simulink model "simple_router"  (R2015a)
settings: Solver=ode45  StartTime=0.0  StopTime=3000  FixedStep=1  RelTol=1e-3
undefined symbols (not defined in the file or in its folder): des, SELECT, T
libraries: simulink x16
(part 3 of 6)

== system simple_router/Router01 ==
  Attribute Function : Subsystem  LoadFcn=des.afb.attributefunction_support(gcb,'LoadFcn');  StartFcn=des.afb.attributefunction_support(gcb,'StartFcn');  mask(Attribute Function){OutputNamePrefix=out_}
      mask prompts: OutputNamePrefix "Prefix name"
      settings: CopyFcn=des.afb.attributefunction_support(gcb,'CopyFcn');  OpenFcn=des.afb.attributefunction_support(gcb,'OpenFcn');  ErrorFcn=des.afb.error_redirect
      mask Help: slhelp(gcbh)
      mask Display: image(des_iconLoad('attribFunction.jpg'),'center');
  Clocked FIFO1 : Subsystem  mask{E=1/F, S=S, F=C}
      mask prompts: E "Clock Period (s)"; S "Standard Deviation"; F "FIFO capacity"
  Clocked FIFO2 : Subsystem  mask{E=1, S=.1, F=8}
      mask prompts: E "Clock Period (s)"; S "Standard Deviation"; F "FIFO capacity"
  Clocked FIFO3 : Subsystem  mask{E=1, S=.1, F=8}
      mask prompts: E "Clock Period (s)"; S "Standard Deviation"; F "FIFO capacity"
  Clocked FIFO4 : Subsystem  mask{E=1, S=.1, F=8}
      mask prompts: E "Clock Period (s)"; S "Standard Deviation"; F "FIFO capacity"
  Clocked FIFO5 : Subsystem  mask{E=1, S=.1, F=8}
      mask prompts: E "Clock Period (s)"; S "Standard Deviation"; F "FIFO capacity"
  Constant : Constant  Value=ME
  Output Switch1 : OutputSwitch  NumberOutputPorts=5  SwitchingCriterion=From attribute  AttributeName=RT  InitialConditionsOpt=on  InitialConditions=5
  Path Combiner : PathCombiner  NumberInputPorts=5  InputPortPrecedence=Equiprobable  InitialSeed=2
  Set Attribute : SetAttribute  AttributeName=ME  AttributeFrom=Signal port  EvaluatedAttributeValue={ []}
  Single Server1 : SingleServer  ServiceTime=D
  DataOut_N : PMIOPort  Port=1  Side=Left
  DataIn_N : PMIOPort  Port=2  Side=Right
  DataIn_W : PMIOPort  Port=3  Side=Left
  DataOut_W : PMIOPort  Port=4  Side=Right
  DataIn_E : PMIOPort  Port=5  Side=Left
  DataOut_E : PMIOPort  Port=6  Side=Right
  DataIn_S : PMIOPort  Port=7  Side=Left
  DataOut_S : PMIOPort  Port=8  Side=Right
  DataIn_NI : PMIOPort  Port=9  Side=Left
  DataOut_NI : PMIOPort  Port=10  Side=Right
  wires:
  Constant/1 -> Set Attribute/1
  connections:
  DataIn_W/RConn1 -- Clocked FIFO2/LConn1
  Clocked FIFO4/LConn1 -- DataIn_E/RConn1
  Clocked FIFO3/LConn1 -- DataIn_S/RConn1
  DataIn_N/RConn1 -- Clocked FIFO1/LConn1
  Clocked FIFO5/LConn1 -- DataIn_NI/RConn1
  Set Attribute/RConn1 -- Attribute Function/LConn1
  Output Switch1/LConn1 -- Single Server1/RConn1
  Single Server1/LConn1 -- Attribute Function/RConn1
  Path Combiner/RConn1 -- Set Attribute/LConn1
  Clocked FIFO1/RConn1 -- Path Combiner/LConn1
  Clocked FIFO2/RConn1 -- Path Combiner/LConn2
  Clocked FIFO4/RConn1 -- Path Combiner/LConn3
  Clocked FIFO3/RConn1 -- Path Combiner/LConn4
  Clocked FIFO5/RConn1 -- Path Combiner/LConn5
  DataOut_N/RConn1 -- Output Switch1/RConn1
  DataOut_W/RConn1 -- Output Switch1/RConn2
  DataOut_E/RConn1 -- Output Switch1/RConn3
  DataOut_S/RConn1 -- Output Switch1/RConn4
  DataOut_NI/RConn1 -- Output Switch1/RConn5

== system simple_router/Router02 ==
  Attribute Function : Subsystem  LoadFcn=des.afb.attributefunction_support(gcb,'LoadFcn');  StartFcn=des.afb.attributefunction_support(gcb,'StartFcn');  mask(Attribute Function){OutputNamePrefix=out_}
      mask prompts: OutputNamePrefix "Prefix name"
      settings: CopyFcn=des.afb.attributefunction_support(gcb,'CopyFcn');  OpenFcn=des.afb.attributefunction_support(gcb,'OpenFcn');  ErrorFcn=des.afb.error_redirect
      mask Help: slhelp(gcbh)
      mask Display: image(des_iconLoad('attribFunction.jpg'),'center');
  Clocked FIFO1 : Subsystem  mask{E=1/F, S=S, F=C}
      mask prompts: E "Clock Period (s)"; S "Standard Deviation"; F "FIFO capacity"
  Clocked FIFO2 : Subsystem  mask{E=1, S=.1, F=8}
      mask prompts: E "Clock Period (s)"; S "Standard Deviation"; F "FIFO capacity"
  Clocked FIFO3 : Subsystem  mask{E=1, S=.1, F=8}
      mask prompts: E "Clock Period (s)"; S "Standard Deviation"; F "FIFO capacity"
  Clocked FIFO4 : Subsystem  mask{E=1, S=.1, F=8}
      mask prompts: E "Clock Period (s)"; S "Standard Deviation"; F "FIFO capacity"
  Clocked FIFO5 : Subsystem  mask{E=1, S=.1, F=8}
      mask prompts: E "Clock Period (s)"; S "Standard Deviation"; F "FIFO capacity"
  Constant : Constant  Value=ME
  Output Switch1 : OutputSwitch  NumberOutputPorts=5  SwitchingCriterion=From attribute  AttributeName=RT  InitialConditionsOpt=on  InitialConditions=5
  Path Combiner : PathCombiner  NumberInputPorts=5  InputPortPrecedence=Equiprobable  InitialSeed=2
  Set Attribute : SetAttribute  AttributeName=ME  AttributeFrom=Signal port  EvaluatedAttributeValue={ []}
  Single Server1 : SingleServer  ServiceTime=D
  DataOut_N : PMIOPort  Port=1  Side=Left
  DataIn_N : PMIOPort  Port=2  Side=Right
  DataIn_W : PMIOPort  Port=3  Side=Left
  DataOut_W : PMIOPort  Port=4  Side=Right
  DataIn_E : PMIOPort  Port=5  Side=Left
  DataOut_E : PMIOPort  Port=6  Side=Right
  DataIn_S : PMIOPort  Port=7  Side=Left
  DataOut_S : PMIOPort  Port=8  Side=Right
  DataIn_NI : PMIOPort  Port=9  Side=Left
  DataOut_NI : PMIOPort  Port=10  Side=Right
  wires:
  Constant/1 -> Set Attribute/1
  connections:
  DataIn_W/RConn1 -- Clocked FIFO2/LConn1
  Clocked FIFO4/LConn1 -- DataIn_E/RConn1
  Clocked FIFO3/LConn1 -- DataIn_S/RConn1
  DataIn_N/RConn1 -- Clocked FIFO1/LConn1
  Clocked FIFO5/LConn1 -- DataIn_NI/RConn1
  Set Attribute/RConn1 -- Attribute Function/LConn1
  Output Switch1/LConn1 -- Single Server1/RConn1
  Single Server1/LConn1 -- Attribute Function/RConn1
  Path Combiner/RConn1 -- Set Attribute/LConn1
  Clocked FIFO1/RConn1 -- Path Combiner/LConn1
  Clocked FIFO2/RConn1 -- Path Combiner/LConn2
  Clocked FIFO4/RConn1 -- Path Combiner/LConn3
  Clocked FIFO3/RConn1 -- Path Combiner/LConn4
  Clocked FIFO5/RConn1 -- Path Combiner/LConn5
  DataOut_N/RConn1 -- Output Switch1/RConn1
  DataOut_W/RConn1 -- Output Switch1/RConn2
  DataOut_E/RConn1 -- Output Switch1/RConn3
  DataOut_S/RConn1 -- Output Switch1/RConn4
  DataOut_NI/RConn1 -- Output Switch1/RConn5

== system simple_router/Router03 ==
  Attribute Function : Subsystem  LoadFcn=des.afb.attributefunction_support(gcb,'LoadFcn');  StartFcn=des.afb.attributefunction_support(gcb,'StartFcn');  mask(Attribute Function){OutputNamePrefix=out_}
      mask prompts: OutputNamePrefix "Prefix name"
      settings: CopyFcn=des.afb.attributefunction_support(gcb,'CopyFcn');  OpenFcn=des.afb.attributefunction_support(gcb,'OpenFcn');  ErrorFcn=des.afb.error_redirect
      mask Help: slhelp(gcbh)
      mask Display: image(des_iconLoad('attribFunction.jpg'),'center');
  Clocked FIFO1 : Subsystem  mask{E=1/F, S=S, F=C}
      mask prompts: E "Clock Period (s)"; S "Standard Deviation"; F "FIFO capacity"
  Clocked FIFO2 : Subsystem  mask{E=1, S=.1, F=8}
      mask prompts: E "Clock Period (s)"; S "Standard Deviation"; F "FIFO capacity"
  Clocked FIFO3 : Subsystem  mask{E=1, S=.1, F=8}
      mask prompts: E "Clock Period (s)"; S "Standard Deviation"; F "FIFO capacity"
  Clocked FIFO4 : Subsystem  mask{E=1, S=.1, F=8}
      mask prompts: E "Clock Period (s)"; S "Standard Deviation"; F "FIFO capacity"
  Clocked FIFO5 : Subsystem  mask{E=1, S=.1, F=8}
      mask prompts: E "Clock Period (s)"; S "Standard Deviation"; F "FIFO capacity"
  Constant : Constant  Value=ME
  Output Switch1 : OutputSwitch  NumberOutputPorts=5  SwitchingCriterion=From attribute  AttributeName=RT  InitialConditionsOpt=on  InitialConditions=5
  Path Combiner : PathCombiner  NumberInputPorts=5  InputPortPrecedence=Equiprobable  InitialSeed=2
  Set Attribute : SetAttribute  AttributeName=ME  AttributeFrom=Signal port  EvaluatedAttributeValue={ []}
  Single Server1 : SingleServer  ServiceTime=D
  DataOut_N : PMIOPort  Port=1  Side=Left
  DataIn_N : PMIOPort  Port=2  Side=Right
  DataIn_W : PMIOPort  Port=3  Side=Left
  DataOut_W : PMIOPort  Port=4  Side=Right
  DataIn_E : PMIOPort  Port=5  Side=Left
  DataOut_E : PMIOPort  Port=6  Side=Right
  DataIn_S : PMIOPort  Port=7  Side=Left
  DataOut_S : PMIOPort  Port=8  Side=Right
  DataIn_NI : PMIOPort  Port=9  Side=Left
  DataOut_NI : PMIOPort  Port=10  Side=Right
  wires:
  Constant/1 -> Set Attribute/1
  connections:
  DataIn_W/RConn1 -- Clocked FIFO2/LConn1
  Clocked FIFO4/LConn1 -- DataIn_E/RConn1
  Clocked FIFO3/LConn1 -- DataIn_S/RConn1
  DataIn_N/RConn1 -- Clocked FIFO1/LConn1
  Clocked FIFO5/LConn1 -- DataIn_NI/RConn1
  Set Attribute/RConn1 -- Attribute Function/LConn1
  Output Switch1/LConn1 -- Single Server1/RConn1
  Single Server1/LConn1 -- Attribute Function/RConn1
  Path Combiner/RConn1 -- Set Attribute/LConn1
  Clocked FIFO1/RConn1 -- Path Combiner/LConn1
  Clocked FIFO2/RConn1 -- Path Combiner/LConn2
  Clocked FIFO4/RConn1 -- Path Combiner/LConn3
  Clocked FIFO3/RConn1 -- Path Combiner/LConn4
  Clocked FIFO5/RConn1 -- Path Combiner/LConn5
  DataOut_N/RConn1 -- Output Switch1/RConn1
  DataOut_W/RConn1 -- Output Switch1/RConn2
  DataOut_E/RConn1 -- Output Switch1/RConn3
  DataOut_S/RConn1 -- Output Switch1/RConn4
  DataOut_NI/RConn1 -- Output Switch1/RConn5

== system simple_router/Router09 ==
  Attribute Function : Subsystem  LoadFcn=des.afb.attributefunction_support(gcb,'LoadFcn');  StartFcn=des.afb.attributefunction_support(gcb,'StartFcn');  mask(Attribute Function){OutputNamePrefix=out_}
      mask prompts: OutputNamePrefix "Prefix name"
      settings: CopyFcn=des.afb.attributefunction_support(gcb,'CopyFcn');  OpenFcn=des.afb.attributefunction_support(gcb,'OpenFcn');  ErrorFcn=des.afb.error_redirect
      mask Help: slhelp(gcbh)
      mask Display: image(des_iconLoad('attribFunction.jpg'),'center');
  Clocked FIFO1 : Subsystem  mask{E=1/F, S=S, F=C}
      mask prompts: E "Clock Period (s)"; S "Standard Deviation"; F "FIFO capacity"
  Clocked FIFO2 : Subsystem  mask{E=1, S=.1, F=8}
      mask prompts: E "Clock Period (s)"; S "Standard Deviation"; F "FIFO capacity"
  Clocked FIFO3 : Subsystem  mask{E=1, S=.1, F=8}
      mask prompts: E "Clock Period (s)"; S "Standard Deviation"; F "FIFO capacity"
  Clocked FIFO4 : Subsystem  mask{E=1, S=.1, F=8}
      mask prompts: E "Clock Period (s)"; S "Standard Deviation"; F "FIFO capacity"
  Clocked FIFO5 : Subsystem  mask{E=1, S=.1, F=8}
      mask prompts: E "Clock Period (s)"; S "Standard Deviation"; F "FIFO capacity"
  Constant : Constant  Value=ME
  Output Switch1 : OutputSwitch  NumberOutputPorts=5  SwitchingCriterion=From attribute  AttributeName=RT  InitialConditionsOpt=on  InitialConditions=5
  Path Combiner : PathCombiner  NumberInputPorts=5  InputPortPrecedence=Equiprobable  InitialSeed=2
  Set Attribute : SetAttribute  AttributeName=ME  AttributeFrom=Signal port  EvaluatedAttributeValue={ []}
  Single Server1 : SingleServer  ServiceTime=D
  DataOut_N : PMIOPort  Port=1  Side=Left
  DataIn_N : PMIOPort  Port=2  Side=Right
  DataIn_W : PMIOPort  Port=3  Side=Left
  DataOut_W : PMIOPort  Port=4  Side=Right
  DataIn_E : PMIOPort  Port=5  Side=Left
  DataOut_E : PMIOPort  Port=6  Side=Right
  DataIn_S : PMIOPort  Port=7  Side=Left
  DataOut_S : PMIOPort  Port=8  Side=Right
  DataIn_NI : PMIOPort  Port=9  Side=Left
  DataOut_NI : PMIOPort  Port=10  Side=Right
  wires:
  Constant/1 -> Set Attribute/1
  connections:
  DataIn_W/RConn1 -- Clocked FIFO2/LConn1
  Clocked FIFO4/LConn1 -- DataIn_E/RConn1
  Clocked FIFO3/LConn1 -- DataIn_S/RConn1
  DataIn_N/RConn1 -- Clocked FIFO1/LConn1
  Clocked FIFO5/LConn1 -- DataIn_NI/RConn1
  Set Attribute/RConn1 -- Attribute Function/LConn1
  Output Switch1/LConn1 -- Single Server1/RConn1
  Single Server1/LConn1 -- Attribute Function/RConn1
  Path Combiner/RConn1 -- Set Attribute/LConn1
  Clocked FIFO1/RConn1 -- Path Combiner/LConn1
  Clocked FIFO2/RConn1 -- Path Combiner/LConn2
  Clocked FIFO4/RConn1 -- Path Combiner/LConn3
  Clocked FIFO3/RConn1 -- Path Combiner/LConn4
  Clocked FIFO5/RConn1 -- Path Combiner/LConn5
  DataOut_N/RConn1 -- Output Switch1/RConn1
  DataOut_W/RConn1 -- Output Switch1/RConn2
  DataOut_E/RConn1 -- Output Switch1/RConn3
  DataOut_S/RConn1 -- Output Switch1/RConn4
  DataOut_NI/RConn1 -- Output Switch1/RConn5

== system simple_router/Router10 ==
  Attribute Function : Subsystem  LoadFcn=des.afb.attributefunction_support(gcb,'LoadFcn');  StartFcn=des.afb.attributefunction_support(gcb,'StartFcn');  mask(Attribute Function){OutputNamePrefix=out_}
      mask prompts: OutputNamePrefix "Prefix name"
      settings: CopyFcn=des.afb.attributefunction_support(gcb,'CopyFcn');  OpenFcn=des.afb.attributefunction_support(gcb,'OpenFcn');  ErrorFcn=des.afb.error_redirect
      mask Help: slhelp(gcbh)
      mask Display: image(des_iconLoad('attribFunction.jpg'),'center');
  Clocked FIFO1 : Subsystem  mask{E=1/F, S=S, F=C}
      mask prompts: E "Clock Period (s)"; S "Standard Deviation"; F "FIFO capacity"
  Clocked FIFO2 : Subsystem  mask{E=1, S=.1, F=8}
      mask prompts: E "Clock Period (s)"; S "Standard Deviation"; F "FIFO capacity"
  Clocked FIFO3 : Subsystem  mask{E=1, S=.1, F=8}
      mask prompts: E "Clock Period (s)"; S "Standard Deviation"; F "FIFO capacity"
  Clocked FIFO4 : Subsystem  mask{E=1, S=.1, F=8}
      mask prompts: E "Clock Period (s)"; S "Standard Deviation"; F "FIFO capacity"
  Clocked FIFO5 : Subsystem  mask{E=1, S=.1, F=8}
      mask prompts: E "Clock Period (s)"; S "Standard Deviation"; F "FIFO capacity"
  Constant : Constant  Value=ME
  Output Switch1 : OutputSwitch  NumberOutputPorts=5  SwitchingCriterion=From attribute  AttributeName=RT  InitialConditionsOpt=on  InitialConditions=5
  Path Combiner : PathCombiner  NumberInputPorts=5  InputPortPrecedence=Equiprobable  InitialSeed=2
  Set Attribute : SetAttribute  AttributeName=ME  AttributeFrom=Signal port  EvaluatedAttributeValue={ []}
  Single Server1 : SingleServer  ServiceTime=D
  DataOut_N : PMIOPort  Port=1  Side=Left
  DataIn_N : PMIOPort  Port=2  Side=Right
  DataIn_W : PMIOPort  Port=3  Side=Left
  DataOut_W : PMIOPort  Port=4  Side=Right
  DataIn_E : PMIOPort  Port=5  Side=Left
  DataOut_E : PMIOPort  Port=6  Side=Right
  DataIn_S : PMIOPort  Port=7  Side=Left
  DataOut_S : PMIOPort  Port=8  Side=Right
  DataIn_NI : PMIOPort  Port=9  Side=Left
  DataOut_NI : PMIOPort  Port=10  Side=Right
  wires:
  Constant/1 -> Set Attribute/1
  connections:
  DataIn_W/RConn1 -- Clocked FIFO2/LConn1
  Clocked FIFO4/LConn1 -- DataIn_E/RConn1
  Clocked FIFO3/LConn1 -- DataIn_S/RConn1
  DataIn_N/RConn1 -- Clocked FIFO1/LConn1
  Clocked FIFO5/LConn1 -- DataIn_NI/RConn1
  Set Attribute/RConn1 -- Attribute Function/LConn1
  Output Switch1/LConn1 -- Single Server1/RConn1
  Single Server1/LConn1 -- Attribute Function/RConn1
  Path Combiner/RConn1 -- Set Attribute/LConn1
  Clocked FIFO1/RConn1 -- Path Combiner/LConn1
  Clocked FIFO2/RConn1 -- Path Combiner/LConn2
  Clocked FIFO4/RConn1 -- Path Combiner/LConn3
  Clocked FIFO3/RConn1 -- Path Combiner/LConn4
  Clocked FIFO5/RConn1 -- Path Combiner/LConn5
  DataOut_N/RConn1 -- Output Switch1/RConn1
  DataOut_W/RConn1 -- Output Switch1/RConn2
  DataOut_E/RConn1 -- Output Switch1/RConn3
  DataOut_S/RConn1 -- Output Switch1/RConn4
  DataOut_NI/RConn1 -- Output Switch1/RConn5

== system simple_router/Router11 ==
  Attribute Function : Subsystem  LoadFcn=des.afb.attributefunction_support(gcb,'LoadFcn');  StartFcn=des.afb.attributefunction_support(gcb,'StartFcn');  mask(Attribute Function){OutputNamePrefix=out_}
      mask prompts: OutputNamePrefix "Prefix name"
      settings: CopyFcn=des.afb.attributefunction_support(gcb,'CopyFcn');  OpenFcn=des.afb.attributefunction_support(gcb,'OpenFcn');  ErrorFcn=des.afb.error_redirect
      mask Help: slhelp(gcbh)
      mask Display: image(des_iconLoad('attribFunction.jpg'),'center');
  Clocked FIFO1 : Subsystem  mask{E=1/F, S=S, F=C}
      mask prompts: E "Clock Period (s)"; S "Standard Deviation"; F "FIFO capacity"
  Clocked FIFO2 : Subsystem  mask{E=1, S=.1, F=8}
      mask prompts: E "Clock Period (s)"; S "Standard Deviation"; F "FIFO capacity"
  Clocked FIFO3 : Subsystem  mask{E=1, S=.1, F=8}
      mask prompts: E "Clock Period (s)"; S "Standard Deviation"; F "FIFO capacity"
  Clocked FIFO4 : Subsystem  mask{E=1, S=.1, F=8}
      mask prompts: E "Clock Period (s)"; S "Standard Deviation"; F "FIFO capacity"
  Clocked FIFO5 : Subsystem  mask{E=1, S=.1, F=8}
      mask prompts: E "Clock Period (s)"; S "Standard Deviation"; F "FIFO capacity"
  Constant : Constant  Value=ME
  Output Switch1 : OutputSwitch  NumberOutputPorts=5  SwitchingCriterion=From attribute  AttributeName=RT  InitialConditionsOpt=on  InitialConditions=5
  Path Combiner : PathCombiner  NumberInputPorts=5  InputPortPrecedence=Equiprobable  InitialSeed=2
  Set Attribute : SetAttribute  AttributeName=ME  AttributeFrom=Signal port  EvaluatedAttributeValue={ []}
  Single Server1 : SingleServer  ServiceTime=D
  DataOut_N : PMIOPort  Port=1  Side=Left
  DataIn_N : PMIOPort  Port=2  Side=Right
  DataIn_W : PMIOPort  Port=3  Side=Left
  DataOut_W : PMIOPort  Port=4  Side=Right
  DataIn_E : PMIOPort  Port=5  Side=Left
  DataOut_E : PMIOPort  Port=6  Side=Right
  DataIn_S : PMIOPort  Port=7  Side=Left
  DataOut_S : PMIOPort  Port=8  Side=Right
  DataIn_NI : PMIOPort  Port=9  Side=Left
  DataOut_NI : PMIOPort  Port=10  Side=Right
  wires:
  Constant/1 -> Set Attribute/1
  connections:
  DataIn_W/RConn1 -- Clocked FIFO2/LConn1
  Clocked FIFO4/LConn1 -- DataIn_E/RConn1
  Clocked FIFO3/LConn1 -- DataIn_S/RConn1
  DataIn_N/RConn1 -- Clocked FIFO1/LConn1
  Clocked FIFO5/LConn1 -- DataIn_NI/RConn1
  Set Attribute/RConn1 -- Attribute Function/LConn1
  Output Switch1/LConn1 -- Single Server1/RConn1
  Single Server1/LConn1 -- Attribute Function/RConn1
  Path Combiner/RConn1 -- Set Attribute/LConn1
  Clocked FIFO1/RConn1 -- Path Combiner/LConn1
  Clocked FIFO2/RConn1 -- Path Combiner/LConn2
  Clocked FIFO4/RConn1 -- Path Combiner/LConn3
  Clocked FIFO3/RConn1 -- Path Combiner/LConn4
  Clocked FIFO5/RConn1 -- Path Combiner/LConn5
  DataOut_N/RConn1 -- Output Switch1/RConn1
  DataOut_W/RConn1 -- Output Switch1/RConn2
  DataOut_E/RConn1 -- Output Switch1/RConn3
  DataOut_S/RConn1 -- Output Switch1/RConn4
  DataOut_NI/RConn1 -- Output Switch1/RConn5

== system simple_router/Router12 ==
  Attribute Function : Subsystem  LoadFcn=des.afb.attributefunction_support(gcb,'LoadFcn');  StartFcn=des.afb.attributefunction_support(gcb,'StartFcn');  mask(Attribute Function){OutputNamePrefix=out_}
      mask prompts: OutputNamePrefix "Prefix name"
      settings: CopyFcn=des.afb.attributefunction_support(gcb,'CopyFcn');  OpenFcn=des.afb.attributefunction_support(gcb,'OpenFcn');  ErrorFcn=des.afb.error_redirect
      mask Help: slhelp(gcbh)
      mask Display: image(des_iconLoad('attribFunction.jpg'),'center');
  Clocked FIFO1 : Subsystem  mask{E=1/F, S=S, F=C}
      mask prompts: E "Clock Period (s)"; S "Standard Deviation"; F "FIFO capacity"
  Clocked FIFO2 : Subsystem  mask{E=1, S=.1, F=8}
      mask prompts: E "Clock Period (s)"; S "Standard Deviation"; F "FIFO capacity"
  Clocked FIFO3 : Subsystem  mask{E=1, S=.1, F=8}
      mask prompts: E "Clock Period (s)"; S "Standard Deviation"; F "FIFO capacity"
  Clocked FIFO4 : Subsystem  mask{E=1, S=.1, F=8}
      mask prompts: E "Clock Period (s)"; S "Standard Deviation"; F "FIFO capacity"
  Clocked FIFO5 : Subsystem  mask{E=1, S=.1, F=8}
      mask prompts: E "Clock Period (s)"; S "Standard Deviation"; F "FIFO capacity"
  Constant : Constant  Value=ME
  Output Switch1 : OutputSwitch  NumberOutputPorts=5  SwitchingCriterion=From attribute  AttributeName=RT  InitialConditionsOpt=on  InitialConditions=5
  Path Combiner : PathCombiner  NumberInputPorts=5  InputPortPrecedence=Equiprobable  InitialSeed=2
  Set Attribute : SetAttribute  AttributeName=ME  AttributeFrom=Signal port  StatNumberDeparted=on  EvaluatedAttributeValue={ []}
  Single Server1 : SingleServer  ServiceTime=D
  DataOut_N : PMIOPort  Port=1  Side=Left
  DataIn_N : PMIOPort  Port=2  Side=Right
  DataIn_W : PMIOPort  Port=3  Side=Left
  DataOut_W : PMIOPort  Port=4  Side=Right
  DataIn_E : PMIOPort  Port=5  Side=Left
  DataOut_E : PMIOPort  Port=6  Side=Right
  DataIn_S : PMIOPort  Port=7  Side=Left
  DataOut_S : PMIOPort  Port=8  Side=Right
  DataIn_NI : PMIOPort  Port=9  Side=Left
  DataOut_NI : PMIOPort  Port=10  Side=Right
  wires:
  Constant/1 -> Set Attribute/1
  connections:
  DataIn_W/RConn1 -- Clocked FIFO2/LConn1
  Clocked FIFO4/LConn1 -- DataIn_E/RConn1
  Clocked FIFO3/LConn1 -- DataIn_S/RConn1
  DataIn_N/RConn1 -- Clocked FIFO1/LConn1
  Clocked FIFO5/LConn1 -- DataIn_NI/RConn1
  Set Attribute/RConn1 -- Attribute Function/LConn1
  Output Switch1/LConn1 -- Single Server1/RConn1
  Single Server1/LConn1 -- Attribute Function/RConn1
  Path Combiner/RConn1 -- Set Attribute/LConn1
  Clocked FIFO1/RConn1 -- Path Combiner/LConn1
  Clocked FIFO2/RConn1 -- Path Combiner/LConn2
  Clocked FIFO4/RConn1 -- Path Combiner/LConn3
  Clocked FIFO3/RConn1 -- Path Combiner/LConn4
  Clocked FIFO5/RConn1 -- Path Combiner/LConn5
  DataOut_N/RConn1 -- Output Switch1/RConn1
  DataOut_W/RConn1 -- Output Switch1/RConn2
  DataOut_E/RConn1 -- Output Switch1/RConn3
  DataOut_S/RConn1 -- Output Switch1/RConn4
  DataOut_NI/RConn1 -- Output Switch1/RConn5

== system simple_router/Router13 ==
  Attribute Function : Subsystem  LoadFcn=des.afb.attributefunction_support(gcb,'LoadFcn');  StartFcn=des.afb.attributefunction_support(gcb,'StartFcn');  mask(Attribute Function){OutputNamePrefix=out_}
      mask prompts: OutputNamePrefix "Prefix name"
      settings: CopyFcn=des.afb.attributefunction_support(gcb,'CopyFcn');  OpenFcn=des.afb.attributefunction_support(gcb,'OpenFcn');  ErrorFcn=des.afb.error_redirect
      mask Help: slhelp(gcbh)
      mask Display: image(des_iconLoad('attribFunction.jpg'),'center');
  Clocked FIFO1 : Subsystem  mask{E=1/F, S=S, F=C}
      mask prompts: E "Clock Period (s)"; S "Standard Deviation"; F "FIFO capacity"
  Clocked FIFO2 : Subsystem  mask{E=1, S=.1, F=8}
      mask prompts: E "Clock Period (s)"; S "Standard Deviation"; F "FIFO capacity"
  Clocked FIFO3 : Subsystem  mask{E=1, S=.1, F=8}
      mask prompts: E "Clock Period (s)"; S "Standard Deviation"; F "FIFO capacity"
  Clocked FIFO4 : Subsystem  mask{E=1, S=.1, F=8}
      mask prompts: E "Clock Period (s)"; S "Standard Deviation"; F "FIFO capacity"
  Clocked FIFO5 : Subsystem  mask{E=1, S=.1, F=8}
      mask prompts: E "Clock Period (s)"; S "Standard Deviation"; F "FIFO capacity"
  Constant : Constant  Value=ME
  Output Switch1 : OutputSwitch  NumberOutputPorts=5  SwitchingCriterion=From attribute  AttributeName=RT  InitialConditionsOpt=on  InitialConditions=5
  Path Combiner : PathCombiner  NumberInputPorts=5  InputPortPrecedence=Equiprobable  InitialSeed=2
  Set Attribute : SetAttribute  AttributeName=ME  AttributeFrom=Signal port  EvaluatedAttributeValue={ []}
  Single Server1 : SingleServer  ServiceTime=D
  DataOut_N : PMIOPort  Port=1  Side=Left
  DataIn_N : PMIOPort  Port=2  Side=Right
  DataIn_W : PMIOPort  Port=3  Side=Left
  DataOut_W : PMIOPort  Port=4  Side=Right
  DataIn_E : PMIOPort  Port=5  Side=Left
  DataOut_E : PMIOPort  Port=6  Side=Right
  DataIn_S : PMIOPort  Port=7  Side=Left
  DataOut_S : PMIOPort  Port=8  Side=Right
  DataIn_NI : PMIOPort  Port=9  Side=Left
  DataOut_NI : PMIOPort  Port=10  Side=Right
  wires:
  Constant/1 -> Set Attribute/1
  connections:
  DataIn_W/RConn1 -- Clocked FIFO2/LConn1
  Clocked FIFO4/LConn1 -- DataIn_E/RConn1
  Clocked FIFO3/LConn1 -- DataIn_S/RConn1
  DataIn_N/RConn1 -- Clocked FIFO1/LConn1
  Clocked FIFO5/LConn1 -- DataIn_NI/RConn1
  Set Attribute/RConn1 -- Attribute Function/LConn1
  Output Switch1/LConn1 -- Single Server1/RConn1
  Single Server1/LConn1 -- Attribute Function/RConn1
  Path Combiner/RConn1 -- Set Attribute/LConn1
  Clocked FIFO1/RConn1 -- Path Combiner/LConn1
  Clocked FIFO2/RConn1 -- Path Combiner/LConn2
  Clocked FIFO4/RConn1 -- Path Combiner/LConn3
  Clocked FIFO3/RConn1 -- Path Combiner/LConn4
  Clocked FIFO5/RConn1 -- Path Combiner/LConn5
  DataOut_N/RConn1 -- Output Switch1/RConn1
  DataOut_W/RConn1 -- Output Switch1/RConn2
  DataOut_E/RConn1 -- Output Switch1/RConn3
  DataOut_S/RConn1 -- Output Switch1/RConn4
  DataOut_NI/RConn1 -- Output Switch1/RConn5

== system simple_router/Router20 ==
  Attribute Function : Subsystem  LoadFcn=des.afb.attributefunction_support(gcb,'LoadFcn');  StartFcn=des.afb.attributefunction_support(gcb,'StartFcn');  mask(Attribute Function){OutputNamePrefix=out_}
      mask prompts: OutputNamePrefix "Prefix name"
      settings: CopyFcn=des.afb.attributefunction_support(gcb,'CopyFcn');  OpenFcn=des.afb.attributefunction_support(gcb,'OpenFcn');  ErrorFcn=des.afb.error_redirect
      mask Help: slhelp(gcbh)
      mask Display: image(des_iconLoad('attribFunction.jpg'),'center');
  Clocked FIFO1 : Subsystem  mask{E=1/F, S=S, F=C}
      mask prompts: E "Clock Period (s)"; S "Standard Deviation"; F "FIFO capacity"
  Clocked FIFO2 : Subsystem  mask{E=1, S=.1, F=8}
      mask prompts: E "Clock Period (s)"; S "Standard Deviation"; F "FIFO capacity"
  Clocked FIFO3 : Subsystem  mask{E=1, S=.1, F=8}
      mask prompts: E "Clock Period (s)"; S "Standard Deviation"; F "FIFO capacity"
  Clocked FIFO4 : Subsystem  mask{E=1, S=.1, F=8}
      mask prompts: E "Clock Period (s)"; S "Standard Deviation"; F "FIFO capacity"
  Clocked FIFO5 : Subsystem  mask{E=1, S=.1, F=8}
      mask prompts: E "Clock Period (s)"; S "Standard Deviation"; F "FIFO capacity"
  Constant : Constant  Value=ME
  Output Switch1 : OutputSwitch  NumberOutputPorts=5  SwitchingCriterion=From attribute  AttributeName=RT  InitialConditionsOpt=on  InitialConditions=5
  Path Combiner : PathCombiner  NumberInputPorts=5  InputPortPrecedence=Equiprobable  InitialSeed=2
  Set Attribute : SetAttribute  AttributeName=ME  AttributeFrom=Signal port  EvaluatedAttributeValue={ []}
  Single Server1 : SingleServer  ServiceTime=D
  DataOut_N : PMIOPort  Port=1  Side=Left
  DataIn_N : PMIOPort  Port=2  Side=Right
  DataIn_W : PMIOPort  Port=3  Side=Left
  DataOut_W : PMIOPort  Port=4  Side=Right
  DataIn_E : PMIOPort  Port=5  Side=Left
  DataOut_E : PMIOPort  Port=6  Side=Right
  DataIn_S : PMIOPort  Port=7  Side=Left
  DataOut_S : PMIOPort  Port=8  Side=Right
  DataIn_NI : PMIOPort  Port=9  Side=Left
  DataOut_NI : PMIOPort  Port=10  Side=Right
  wires:
  Constant/1 -> Set Attribute/1
  connections:
  DataIn_W/RConn1 -- Clocked FIFO2/LConn1
  Clocked FIFO4/LConn1 -- DataIn_E/RConn1
  Clocked FIFO3/LConn1 -- DataIn_S/RConn1
  DataIn_N/RConn1 -- Clocked FIFO1/LConn1
  Clocked FIFO5/LConn1 -- DataIn_NI/RConn1
  Set Attribute/RConn1 -- Attribute Function/LConn1
  Output Switch1/LConn1 -- Single Server1/RConn1
  Single Server1/LConn1 -- Attribute Function/RConn1
  Path Combiner/RConn1 -- Set Attribute/LConn1
  Clocked FIFO1/RConn1 -- Path Combiner/LConn1
  Clocked FIFO2/RConn1 -- Path Combiner/LConn2
  Clocked FIFO4/RConn1 -- Path Combiner/LConn3
  Clocked FIFO3/RConn1 -- Path Combiner/LConn4
  Clocked FIFO5/RConn1 -- Path Combiner/LConn5
  DataOut_N/RConn1 -- Output Switch1/RConn1
  DataOut_W/RConn1 -- Output Switch1/RConn2
  DataOut_E/RConn1 -- Output Switch1/RConn3
  DataOut_S/RConn1 -- Output Switch1/RConn4
  DataOut_NI/RConn1 -- Output Switch1/RConn5

== system simple_router/Router22 ==
  Attribute Function : Subsystem  LoadFcn=des.afb.attributefunction_support(gcb,'LoadFcn');  StartFcn=des.afb.attributefunction_support(gcb,'StartFcn');  mask(Attribute Function){OutputNamePrefix=out_}
      mask prompts: OutputNamePrefix "Prefix name"
      settings: CopyFcn=des.afb.attributefunction_support(gcb,'CopyFcn');  OpenFcn=des.afb.attributefunction_support(gcb,'OpenFcn');  ErrorFcn=des.afb.error_redirect
      mask Help: slhelp(gcbh)
      mask Display: image(des_iconLoad('attribFunction.jpg'),'center');
  Clocked FIFO1 : Subsystem  mask{E=1/F, S=S, F=C}
      mask prompts: E "Clock Period (s)"; S "Standard Deviation"; F "FIFO capacity"
  Clocked FIFO2 : Subsystem  mask{E=1, S=.1, F=8}
      mask prompts: E "Clock Period (s)"; S "Standard Deviation"; F "FIFO capacity"
  Clocked FIFO3 : Subsystem  mask{E=1, S=.1, F=8}
      mask prompts: E "Clock Period (s)"; S "Standard Deviation"; F "FIFO capacity"
  Clocked FIFO4 : Subsystem  mask{E=1, S=.1, F=8}
      mask prompts: E "Clock Period (s)"; S "Standard Deviation"; F "FIFO capacity"
  Clocked FIFO5 : Subsystem  mask{E=1, S=.1, F=8}
      mask prompts: E "Clock Period (s)"; S "Standard Deviation"; F "FIFO capacity"
  Constant : Constant  Value=ME
  Output Switch1 : OutputSwitch  NumberOutputPorts=5  SwitchingCriterion=From attribute  AttributeName=RT  InitialConditionsOpt=on  InitialConditions=5
  Path Combiner : PathCombiner  NumberInputPorts=5  InputPortPrecedence=Equiprobable  InitialSeed=2
  Set Attribute : SetAttribute  AttributeName=ME  AttributeFrom=Signal port  EvaluatedAttributeValue={ []}
  Single Server1 : SingleServer  ServiceTime=D
  DataOut_N : PMIOPort  Port=1  Side=Left
  DataIn_N : PMIOPort  Port=2  Side=Right
  DataIn_W : PMIOPort  Port=3  Side=Left
  DataOut_W : PMIOPort  Port=4  Side=Right
  DataIn_E : PMIOPort  Port=5  Side=Left
  DataOut_E : PMIOPort  Port=6  Side=Right
  DataIn_S : PMIOPort  Port=7  Side=Left
  DataOut_S : PMIOPort  Port=8  Side=Right
  DataIn_NI : PMIOPort  Port=9  Side=Left
  DataOut_NI : PMIOPort  Port=10  Side=Right
  wires:
  Constant/1 -> Set Attribute/1
  connections:
  DataIn_W/RConn1 -- Clocked FIFO2/LConn1
  Clocked FIFO4/LConn1 -- DataIn_E/RConn1
  Clocked FIFO3/LConn1 -- DataIn_S/RConn1
  DataIn_N/RConn1 -- Clocked FIFO1/LConn1
  Clocked FIFO5/LConn1 -- DataIn_NI/RConn1
  Set Attribute/RConn1 -- Attribute Function/LConn1
  Output Switch1/LConn1 -- Single Server1/RConn1
  Single Server1/LConn1 -- Attribute Function/RConn1
  Path Combiner/RConn1 -- Set Attribute/LConn1
  Clocked FIFO1/RConn1 -- Path Combiner/LConn1
  Clocked FIFO2/RConn1 -- Path Combiner/LConn2
  Clocked FIFO4/RConn1 -- Path Combiner/LConn3
  Clocked FIFO3/RConn1 -- Path Combiner/LConn4
  Clocked FIFO5/RConn1 -- Path Combiner/LConn5
  DataOut_N/RConn1 -- Output Switch1/RConn1
  DataOut_W/RConn1 -- Output Switch1/RConn2
  DataOut_E/RConn1 -- Output Switch1/RConn3
  DataOut_S/RConn1 -- Output Switch1/RConn4
  DataOut_NI/RConn1 -- Output Switch1/RConn5

== system simple_router/Router23 ==
  Attribute Function : Subsystem  LoadFcn=des.afb.attributefunction_support(gcb,'LoadFcn');  StartFcn=des.afb.attributefunction_support(gcb,'StartFcn');  mask(Attribute Function){OutputNamePrefix=out_}
      mask prompts: OutputNamePrefix "Prefix name"
      settings: CopyFcn=des.afb.attributefunction_support(gcb,'CopyFcn');  OpenFcn=des.afb.attributefunction_support(gcb,'OpenFcn');  ErrorFcn=des.afb.error_redirect
      mask Help: slhelp(gcbh)
      mask Display: image(des_iconLoad('attribFunction.jpg'),'center');
  Clocked FIFO1 : Subsystem  mask{E=1/F, S=S, F=C}
      mask prompts: E "Clock Period (s)"; S "Standard Deviation"; F "FIFO capacity"
  Clocked FIFO2 : Subsystem  mask{E=1, S=.1, F=8}
      mask prompts: E "Clock Period (s)"; S "Standard Deviation"; F "FIFO capacity"
  Clocked FIFO3 : Subsystem  mask{E=1, S=.1, F=8}
      mask prompts: E "Clock Period (s)"; S "Standard Deviation"; F "FIFO capacity"
  Clocked FIFO4 : Subsystem  mask{E=1, S=.1, F=8}
      mask prompts: E "Clock Period (s)"; S "Standard Deviation"; F "FIFO capacity"
  Clocked FIFO5 : Subsystem  mask{E=1, S=.1, F=8}
      mask prompts: E "Clock Period (s)"; S "Standard Deviation"; F "FIFO capacity"
  Constant : Constant  Value=ME
  Output Switch1 : OutputSwitch  NumberOutputPorts=5  SwitchingCriterion=From attribute  AttributeName=RT  InitialConditionsOpt=on  InitialConditions=5
  Path Combiner : PathCombiner  NumberInputPorts=5  InputPortPrecedence=Equiprobable  InitialSeed=2
  Set Attribute : SetAttribute  AttributeName=ME  AttributeFrom=Signal port  EvaluatedAttributeValue={ []}
  Single Server1 : SingleServer  ServiceTime=D
  DataOut_N : PMIOPort  Port=1  Side=Left
  DataIn_N : PMIOPort  Port=2  Side=Right
  DataIn_W : PMIOPort  Port=3  Side=Left
  DataOut_W : PMIOPort  Port=4  Side=Right
  DataIn_E : PMIOPort  Port=5  Side=Left
  DataOut_E : PMIOPort  Port=6  Side=Right
  DataIn_S : PMIOPort  Port=7  Side=Left
  DataOut_S : PMIOPort  Port=8  Side=Right
  DataIn_NI : PMIOPort  Port=9  Side=Left
  DataOut_NI : PMIOPort  Port=10  Side=Right
  wires:
  Constant/1 -> Set Attribute/1
  connections:
  DataIn_W/RConn1 -- Clocked FIFO2/LConn1
  Clocked FIFO4/LConn1 -- DataIn_E/RConn1
  Clocked FIFO3/LConn1 -- DataIn_S/RConn1
  DataIn_N/RConn1 -- Clocked FIFO1/LConn1
  Clocked FIFO5/LConn1 -- DataIn_NI/RConn1
  Set Attribute/RConn1 -- Attribute Function/LConn1
  Output Switch1/LConn1 -- Single Server1/RConn1
  Single Server1/LConn1 -- Attribute Function/RConn1
  Path Combiner/RConn1 -- Set Attribute/LConn1
  Clocked FIFO1/RConn1 -- Path Combiner/LConn1
  Clocked FIFO2/RConn1 -- Path Combiner/LConn2
  Clocked FIFO4/RConn1 -- Path Combiner/LConn3
  Clocked FIFO3/RConn1 -- Path Combiner/LConn4
  Clocked FIFO5/RConn1 -- Path Combiner/LConn5
  DataOut_N/RConn1 -- Output Switch1/RConn1
  DataOut_W/RConn1 -- Output Switch1/RConn2
  DataOut_E/RConn1 -- Output Switch1/RConn3
  DataOut_S/RConn1 -- Output Switch1/RConn4
  DataOut_NI/RConn1 -- Output Switch1/RConn5

== system simple_router/Router30 ==
  Attribute Function : Subsystem  LoadFcn=des.afb.attributefunction_support(gcb,'LoadFcn');  StartFcn=des.afb.attributefunction_support(gcb,'StartFcn');  mask(Attribute Function){OutputNamePrefix=out_}
      mask prompts: OutputNamePrefix "Prefix name"
      settings: CopyFcn=des.afb.attributefunction_support(gcb,'CopyFcn');  OpenFcn=des.afb.attributefunction_support(gcb,'OpenFcn');  ErrorFcn=des.afb.error_redirect
      mask Help: slhelp(gcbh)
      mask Display: image(des_iconLoad('attribFunction.jpg'),'center');
  Clocked FIFO1 : Subsystem  mask{E=1/F, S=S, F=C}
      mask prompts: E "Clock Period (s)"; S "Standard Deviation"; F "FIFO capacity"
  Clocked FIFO2 : Subsystem  mask{E=1, S=.1, F=8}
      mask prompts: E "Clock Period (s)"; S "Standard Deviation"; F "FIFO capacity"
  Clocked FIFO3 : Subsystem  mask{E=1, S=.1, F=8}
      mask prompts: E "Clock Period (s)"; S "Standard Deviation"; F "FIFO capacity"
  Clocked FIFO4 : Subsystem  mask{E=1, S=.1, F=8}
      mask prompts: E "Clock Period (s)"; S "Standard Deviation"; F "FIFO capacity"
  Clocked FIFO5 : Subsystem  mask{E=1, S=.1, F=8}
      mask prompts: E "Clock Period (s)"; S "Standard Deviation"; F "FIFO capacity"
  Constant : Constant  Value=ME
  Output Switch1 : OutputSwitch  NumberOutputPorts=5  SwitchingCriterion=From attribute  AttributeName=RT  InitialConditionsOpt=on  InitialConditions=5
  Path Combiner : PathCombiner  NumberInputPorts=5  InputPortPrecedence=Equiprobable  InitialSeed=2
  Set Attribute : SetAttribute  AttributeName=ME  AttributeFrom=Signal port  EvaluatedAttributeValue={ []}
  Single Server1 : SingleServer  ServiceTime=D
  DataOut_N : PMIOPort  Port=1  Side=Left
  DataIn_N : PMIOPort  Port=2  Side=Right
  DataIn_W : PMIOPort  Port=3  Side=Left
  DataOut_W : PMIOPort  Port=4  Side=Right
  DataIn_E : PMIOPort  Port=5  Side=Left
  DataOut_E : PMIOPort  Port=6  Side=Right
  DataIn_S : PMIOPort  Port=7  Side=Left
  DataOut_S : PMIOPort  Port=8  Side=Right
  DataIn_NI : PMIOPort  Port=9  Side=Left
  DataOut_NI : PMIOPort  Port=10  Side=Right
  wires:
  Constant/1 -> Set Attribute/1
  connections:
  DataIn_W/RConn1 -- Clocked FIFO2/LConn1
  Clocked FIFO4/LConn1 -- DataIn_E/RConn1
  Clocked FIFO3/LConn1 -- DataIn_S/RConn1
  DataIn_N/RConn1 -- Clocked FIFO1/LConn1
  Clocked FIFO5/LConn1 -- DataIn_NI/RConn1
  Set Attribute/RConn1 -- Attribute Function/LConn1
  Output Switch1/LConn1 -- Single Server1/RConn1
  Single Server1/LConn1 -- Attribute Function/RConn1
  Path Combiner/RConn1 -- Set Attribute/LConn1
  Clocked FIFO1/RConn1 -- Path Combiner/LConn1
  Clocked FIFO2/RConn1 -- Path Combiner/LConn2
  Clocked FIFO4/RConn1 -- Path Combiner/LConn3
  Clocked FIFO3/RConn1 -- Path Combiner/LConn4
  Clocked FIFO5/RConn1 -- Path Combiner/LConn5
  DataOut_N/RConn1 -- Output Switch1/RConn1
  DataOut_W/RConn1 -- Output Switch1/RConn2
  DataOut_E/RConn1 -- Output Switch1/RConn3
  DataOut_S/RConn1 -- Output Switch1/RConn4
  DataOut_NI/RConn1 -- Output Switch1/RConn5

== system simple_router/Router31 ==
  Attribute Function : Subsystem  LoadFcn=des.afb.attributefunction_support(gcb,'LoadFcn');  StartFcn=des.afb.attributefunction_support(gcb,'StartFcn');  mask(Attribute Function){OutputNamePrefix=out_}
      mask prompts: OutputNamePrefix "Prefix name"
      settings: CopyFcn=des.afb.attributefunction_support(gcb,'CopyFcn');  OpenFcn=des.afb.attributefunction_support(gcb,'OpenFcn');  ErrorFcn=des.afb.error_redirect
      mask Help: slhelp(gcbh)
      mask Display: image(des_iconLoad('attribFunction.jpg'),'center');
  Clocked FIFO1 : Subsystem  mask{E=1/F, S=S, F=C}
      mask prompts: E "Clock Period (s)"; S "Standard Deviation"; F "FIFO capacity"
  Clocked FIFO2 : Subsystem  mask{E=1, S=.1, F=8}
      mask prompts: E "Clock Period (s)"; S "Standard Deviation"; F "FIFO capacity"
  Clocked FIFO3 : Subsystem  mask{E=1, S=.1, F=8}
      mask prompts: E "Clock Period (s)"; S "Standard Deviation"; F "FIFO capacity"
  Clocked FIFO4 : Subsystem  mask{E=1, S=.1, F=8}
      mask prompts: E "Clock Period (s)"; S "Standard Deviation"; F "FIFO capacity"
  Clocked FIFO5 : Subsystem  mask{E=1, S=.1, F=8}
      mask prompts: E "Clock Period (s)"; S "Standard Deviation"; F "FIFO capacity"
  Constant : Constant  Value=ME
  Output Switch1 : OutputSwitch  NumberOutputPorts=5  SwitchingCriterion=From attribute  AttributeName=RT  InitialConditionsOpt=on  InitialConditions=5
  Path Combiner : PathCombiner  NumberInputPorts=5  InputPortPrecedence=Equiprobable  InitialSeed=2
  Set Attribute : SetAttribute  AttributeName=ME  AttributeFrom=Signal port  EvaluatedAttributeValue={ []}
  Single Server1 : SingleServer  ServiceTime=D
  DataOut_N : PMIOPort  Port=1  Side=Left
  DataIn_N : PMIOPort  Port=2  Side=Right
  DataIn_W : PMIOPort  Port=3  Side=Left
  DataOut_W : PMIOPort  Port=4  Side=Right
  DataIn_E : PMIOPort  Port=5  Side=Left
  DataOut_E : PMIOPort  Port=6  Side=Right
  DataIn_S : PMIOPort  Port=7  Side=Left
  DataOut_S : PMIOPort  Port=8  Side=Right
  DataIn_NI : PMIOPort  Port=9  Side=Left
  DataOut_NI : PMIOPort  Port=10  Side=Right
  wires:
  Constant/1 -> Set Attribute/1
  connections:
  DataIn_W/RConn1 -- Clocked FIFO2/LConn1
  Clocked FIFO4/LConn1 -- DataIn_E/RConn1
  Clocked FIFO3/LConn1 -- DataIn_S/RConn1
  DataIn_N/RConn1 -- Clocked FIFO1/LConn1
  Clocked FIFO5/LConn1 -- DataIn_NI/RConn1
  Set Attribute/RConn1 -- Attribute Function/LConn1
  Output Switch1/LConn1 -- Single Server1/RConn1
  Single Server1/LConn1 -- Attribute Function/RConn1
  Path Combiner/RConn1 -- Set Attribute/LConn1
  Clocked FIFO1/RConn1 -- Path Combiner/LConn1
  Clocked FIFO2/RConn1 -- Path Combiner/LConn2
  Clocked FIFO4/RConn1 -- Path Combiner/LConn3
  Clocked FIFO3/RConn1 -- Path Combiner/LConn4
  Clocked FIFO5/RConn1 -- Path Combiner/LConn5
  DataOut_N/RConn1 -- Output Switch1/RConn1
  DataOut_W/RConn1 -- Output Switch1/RConn2
  DataOut_E/RConn1 -- Output Switch1/RConn3
  DataOut_S/RConn1 -- Output Switch1/RConn4
  DataOut_NI/RConn1 -- Output Switch1/RConn5

== system simple_router/Router32 ==
  Attribute Function : Subsystem  LoadFcn=des.afb.attributefunction_support(gcb,'LoadFcn');  StartFcn=des.afb.attributefunction_support(gcb,'StartFcn');  mask(Attribute Function){OutputNamePrefix=out_}
      mask prompts: OutputNamePrefix "Prefix name"
      settings: CopyFcn=des.afb.attributefunction_support(gcb,'CopyFcn');  OpenFcn=des.afb.attributefunction_support(gcb,'OpenFcn');  ErrorFcn=des.afb.error_redirect
      mask Help: slhelp(gcbh)
      mask Display: image(des_iconLoad('attribFunction.jpg'),'center');
  Clocked FIFO1 : Subsystem  mask{E=1/F, S=S, F=C}
      mask prompts: E "Clock Period (s)"; S "Standard Deviation"; F "FIFO capacity"
  Clocked FIFO2 : Subsystem  mask{E=1, S=.1, F=8}
      mask prompts: E "Clock Period (s)"; S "Standard Deviation"; F "FIFO capacity"
  Clocked FIFO3 : Subsystem  mask{E=1, S=.1, F=8}
      mask prompts: E "Clock Period (s)"; S "Standard Deviation"; F "FIFO capacity"
  Clocked FIFO4 : Subsystem  mask{E=1, S=.1, F=8}
      mask prompts: E "Clock Period (s)"; S "Standard Deviation"; F "FIFO capacity"
  Clocked FIFO5 : Subsystem  mask{E=1, S=.1, F=8}
      mask prompts: E "Clock Period (s)"; S "Standard Deviation"; F "FIFO capacity"
  Constant : Constant  Value=ME
  Output Switch1 : OutputSwitch  NumberOutputPorts=5  SwitchingCriterion=From attribute  AttributeName=RT  InitialConditionsOpt=on  InitialConditions=5
  Path Combiner : PathCombiner  NumberInputPorts=5  InputPortPrecedence=Equiprobable  InitialSeed=2
  Set Attribute : SetAttribute  AttributeName=ME  AttributeFrom=Signal port  EvaluatedAttributeValue={ []}
  Single Server1 : SingleServer  ServiceTime=D
  DataOut_N : PMIOPort  Port=1  Side=Left
  DataIn_N : PMIOPort  Port=2  Side=Right
  DataIn_W : PMIOPort  Port=3  Side=Left
  DataOut_W : PMIOPort  Port=4  Side=Right
  DataIn_E : PMIOPort  Port=5  Side=Left
  DataOut_E : PMIOPort  Port=6  Side=Right
  DataIn_S : PMIOPort  Port=7  Side=Left
  DataOut_S : PMIOPort  Port=8  Side=Right
  DataIn_NI : PMIOPort  Port=9  Side=Left
  DataOut_NI : PMIOPort  Port=10  Side=Right
  wires:
  Constant/1 -> Set Attribute/1
  connections:
  DataIn_W/RConn1 -- Clocked FIFO2/LConn1
  Clocked FIFO4/LConn1 -- DataIn_E/RConn1
  Clocked FIFO3/LConn1 -- DataIn_S/RConn1
  DataIn_N/RConn1 -- Clocked FIFO1/LConn1
  Clocked FIFO5/LConn1 -- DataIn_NI/RConn1
  Set Attribute/RConn1 -- Attribute Function/LConn1
  Output Switch1/LConn1 -- Single Server1/RConn1
  Single Server1/LConn1 -- Attribute Function/RConn1
  Path Combiner/RConn1 -- Set Attribute/LConn1
  Clocked FIFO1/RConn1 -- Path Combiner/LConn1
  Clocked FIFO2/RConn1 -- Path Combiner/LConn2
  Clocked FIFO4/RConn1 -- Path Combiner/LConn3
  Clocked FIFO3/RConn1 -- Path Combiner/LConn4
  Clocked FIFO5/RConn1 -- Path Combiner/LConn5
  DataOut_N/RConn1 -- Output Switch1/RConn1
  DataOut_W/RConn1 -- Output Switch1/RConn2
  DataOut_E/RConn1 -- Output Switch1/RConn3
  DataOut_S/RConn1 -- Output Switch1/RConn4
  DataOut_NI/RConn1 -- Output Switch1/RConn5

== system simple_router/Router33 ==
  Attribute Function : Subsystem  LoadFcn=des.afb.attributefunction_support(gcb,'LoadFcn');  StartFcn=des.afb.attributefunction_support(gcb,'StartFcn');  mask(Attribute Function){OutputNamePrefix=out_}
      mask prompts: OutputNamePrefix "Prefix name"
      settings: CopyFcn=des.afb.attributefunction_support(gcb,'CopyFcn');  OpenFcn=des.afb.attributefunction_support(gcb,'OpenFcn');  ErrorFcn=des.afb.error_redirect
      mask Help: slhelp(gcbh)
      mask Display: image(des_iconLoad('attribFunction.jpg'),'center');
  Clocked FIFO1 : Subsystem  mask{E=1/F, S=S, F=C}
      mask prompts: E "Clock Period (s)"; S "Standard Deviation"; F "FIFO capacity"
  Clocked FIFO2 : Subsystem  mask{E=1, S=.1, F=8}
      mask prompts: E "Clock Period (s)"; S "Standard Deviation"; F "FIFO capacity"
  Clocked FIFO3 : Subsystem  mask{E=1, S=.1, F=8}
      mask prompts: E "Clock Period (s)"; S "Standard Deviation"; F "FIFO capacity"
  Clocked FIFO4 : Subsystem  mask{E=1, S=.1, F=8}
      mask prompts: E "Clock Period (s)"; S "Standard Deviation"; F "FIFO capacity"
  Clocked FIFO5 : Subsystem  mask{E=1, S=.1, F=8}
      mask prompts: E "Clock Period (s)"; S "Standard Deviation"; F "FIFO capacity"
  Constant : Constant  Value=ME
  Output Switch1 : OutputSwitch  NumberOutputPorts=5  SwitchingCriterion=From attribute  AttributeName=RT  InitialConditionsOpt=on  InitialConditions=5
  Path Combiner : PathCombiner  NumberInputPorts=5  InputPortPrecedence=Equiprobable  InitialSeed=2
  Set Attribute : SetAttribute  AttributeName=ME  AttributeFrom=Signal port  EvaluatedAttributeValue={ []}
  Single Server1 : SingleServer  ServiceTime=D
  DataOut_N : PMIOPort  Port=1  Side=Left
  DataIn_N : PMIOPort  Port=2  Side=Right
  DataIn_W : PMIOPort  Port=3  Side=Left
  DataOut_W : PMIOPort  Port=4  Side=Right
  DataIn_E : PMIOPort  Port=5  Side=Left
  DataOut_E : PMIOPort  Port=6  Side=Right
  DataIn_S : PMIOPort  Port=7  Side=Left
  DataOut_S : PMIOPort  Port=8  Side=Right
  DataIn_NI : PMIOPort  Port=9  Side=Left
  DataOut_NI : PMIOPort  Port=10  Side=Right
  wires:
  Constant/1 -> Set Attribute/1
  connections:
  DataIn_W/RConn1 -- Clocked FIFO2/LConn1
  Clocked FIFO4/LConn1 -- DataIn_E/RConn1
  Clocked FIFO3/LConn1 -- DataIn_S/RConn1
  DataIn_N/RConn1 -- Clocked FIFO1/LConn1
  Clocked FIFO5/LConn1 -- DataIn_NI/RConn1
  Set Attribute/RConn1 -- Attribute Function/LConn1
  Output Switch1/LConn1 -- Single Server1/RConn1
  Single Server1/LConn1 -- Attribute Function/RConn1
  Path Combiner/RConn1 -- Set Attribute/LConn1
  Clocked FIFO1/RConn1 -- Path Combiner/LConn1
  Clocked FIFO2/RConn1 -- Path Combiner/LConn2
  Clocked FIFO4/RConn1 -- Path Combiner/LConn3
  Clocked FIFO3/RConn1 -- Path Combiner/LConn4
  Clocked FIFO5/RConn1 -- Path Combiner/LConn5
  DataOut_N/RConn1 -- Output Switch1/RConn1
  DataOut_W/RConn1 -- Output Switch1/RConn2
  DataOut_E/RConn1 -- Output Switch1/RConn3
  DataOut_S/RConn1 -- Output Switch1/RConn4
  DataOut_NI/RConn1 -- Output Switch1/RConn5

== system simple_router/PE1/Create Generator Selection Variable ==
  function : TriggerPort  TriggerType=function-call
  Repeating Sequence Stair : simulink/Sources/Repeating Sequence Stair  OutValues=[0 1].'  tsamp=-1  OutMin=[]  OutMax=[]  OutDataTypeStr=float('double')  OutputDataTypeScalingMode=Specify via dialog  OutDataType=float('double')  ConRadixGroup=Best Precision: Vector-wise  OutScaling=2^-12
  Out1 : Outport
  wires:
  Repeating Sequence Stair/1 -> Out1/1

== system simple_router/PE10/Create Generator Selection Variable ==
  function : TriggerPort  TriggerType=function-call
  Repeating Sequence Stair : simulink/Sources/Repeating Sequence Stair  OutValues=[0 1].'  tsamp=-1  OutMin=[]  OutMax=[]  OutDataTypeStr=float('double')  OutputDataTypeScalingMode=Specify via dialog  OutDataType=float('double')  ConRadixGroup=Best Precision: Vector-wise  OutScaling=2^-12
  Out1 : Outport
  wires:
  Repeating Sequence Stair/1 -> Out1/1

== system simple_router/PE11/Create Generator Selection Variable ==
  function : TriggerPort  TriggerType=function-call
  Repeating Sequence Stair : simulink/Sources/Repeating Sequence Stair  OutValues=[0 1].'  tsamp=-1  OutMin=[]  OutMax=[]  OutDataTypeStr=float('double')  OutputDataTypeScalingMode=Specify via dialog  OutDataType=float('double')  ConRadixGroup=Best Precision: Vector-wise  OutScaling=2^-12
  Out1 : Outport
  wires:
  Repeating Sequence Stair/1 -> Out1/1

== system simple_router/PE12/Create Generator Selection Variable ==
  function : TriggerPort  TriggerType=function-call
  Repeating Sequence Stair : simulink/Sources/Repeating Sequence Stair  OutValues=[0 1].'  tsamp=-1  OutMin=[]  OutMax=[]  OutDataTypeStr=float('double')  OutputDataTypeScalingMode=Specify via dialog  OutDataType=float('double')  ConRadixGroup=Best Precision: Vector-wise  OutScaling=2^-12
  Out1 : Outport
  wires:
  Repeating Sequence Stair/1 -> Out1/1

== system simple_router/PE13/Create Generator Selection Variable ==
  function : TriggerPort  TriggerType=function-call
  Repeating Sequence Stair : simulink/Sources/Repeating Sequence Stair  OutValues=[0 1].'  tsamp=-1  OutMin=[]  OutMax=[]  OutDataTypeStr=float('double')  OutputDataTypeScalingMode=Specify via dialog  OutDataType=float('double')  ConRadixGroup=Best Precision: Vector-wise  OutScaling=2^-12
  Out1 : Outport
  wires:
  Repeating Sequence Stair/1 -> Out1/1

== system simple_router/PE14/Create Generator Selection Variable ==
  function : TriggerPort  TriggerType=function-call
  Repeating Sequence Stair : simulink/Sources/Repeating Sequence Stair  OutValues=[0 1].'  tsamp=-1  OutMin=[]  OutMax=[]  OutDataTypeStr=float('double')  OutputDataTypeScalingMode=Specify via dialog  OutDataType=float('double')  ConRadixGroup=Best Precision: Vector-wise  OutScaling=2^-12
  Out1 : Outport
  wires:
  Repeating Sequence Stair/1 -> Out1/1

== system simple_router/PE15/Create Generator Selection Variable ==
  function : TriggerPort  TriggerType=function-call
  Repeating Sequence Stair : simulink/Sources/Repeating Sequence Stair  OutValues=[0 1].'  tsamp=-1  OutMin=[]  OutMax=[]  OutDataTypeStr=float('double')  OutputDataTypeScalingMode=Specify via dialog  OutDataType=float('double')  ConRadixGroup=Best Precision: Vector-wise  OutScaling=2^-12
  Out1 : Outport
  wires:
  Repeating Sequence Stair/1 -> Out1/1

== system simple_router/PE16/Create Generator Selection Variable ==
  function : TriggerPort  TriggerType=function-call
  Repeating Sequence Stair : simulink/Sources/Repeating Sequence Stair  OutValues=[0 1].'  tsamp=-1  OutMin=[]  OutMax=[]  OutDataTypeStr=float('double')  OutputDataTypeScalingMode=Specify via dialog  OutDataType=float('double')  ConRadixGroup=Best Precision: Vector-wise  OutScaling=2^-12
  Out1 : Outport
  wires:
  Repeating Sequence Stair/1 -> Out1/1

== system simple_router/PE2/Create Generator Selection Variable ==
  function : TriggerPort  TriggerType=function-call
  Repeating Sequence Stair : simulink/Sources/Repeating Sequence Stair  OutValues=[0 1].'  tsamp=-1  OutMin=[]  OutMax=[]  OutDataTypeStr=float('double')  OutputDataTypeScalingMode=Specify via dialog  OutDataType=float('double')  ConRadixGroup=Best Precision: Vector-wise  OutScaling=2^-12
  Out1 : Outport
  wires:
  Repeating Sequence Stair/1 -> Out1/1
